simulink model "decimation_fir"  (Simulink 7.3)
settings: Solver=FixedStepDiscrete  StartTime=0.0  StopTime=3000 * SampleTime  RelTol=1e-3
PreLoadFcn:
  | setup_decimation_fir;
InitFcn:
  | setup_decimation_fir;
values from neighbouring files (symbols this model uses):
  ChanCycleCount = ceil(ChanCount/ChanWireCount)    [setup_decimation_fir.m]
  ChanWireCount = ceil(ChanCount/Period)    [setup_decimation_fir.m]
  ClockRate = ' num2str(ClockRate) '    [setup_decimation_fir.m]
  Period = ClockRate / SampleRate    (= 4)    [setup_decimation_fir.m]
  period_out = Period*Decimation    (= 16)    [setup_decimation_fir.m]
  SampleTime = 1    [setup_decimation_fir.m]
libraries: DSPBABase x8, simulink x7, dspsrcs4 x2
Description:
  | This model shows how to use the DecimatingFIR block to build a 16-channel decimate by 5 49-tap FIR filter. The target system clock frequency is 240 MHz.
  | The model will generate RTL that can be used in the third party tools.
  | The parameters for the system can be modified in the file setup_demo_fird.m which can be accessed from the Edit Params icon.
settings Model: Creator=sichou  LastModifiedBy=xdong
settings OptimizationCC: InitFltsAndDblsToZero=on
settings DebuggingCC: SaveWithParameterizedLinksMsg=none  SignalResolutionControl=TryResolveAllWithWarning  MultiTaskDSMMsg=warning  MultiTaskCondExecSysMsg=none  StrictBusMsg=None
settings RTWCC: IncludeERTFirstTime=on
settings GRTTargetCC: TargetFcnLib=ansi_tfl_tmw.mat

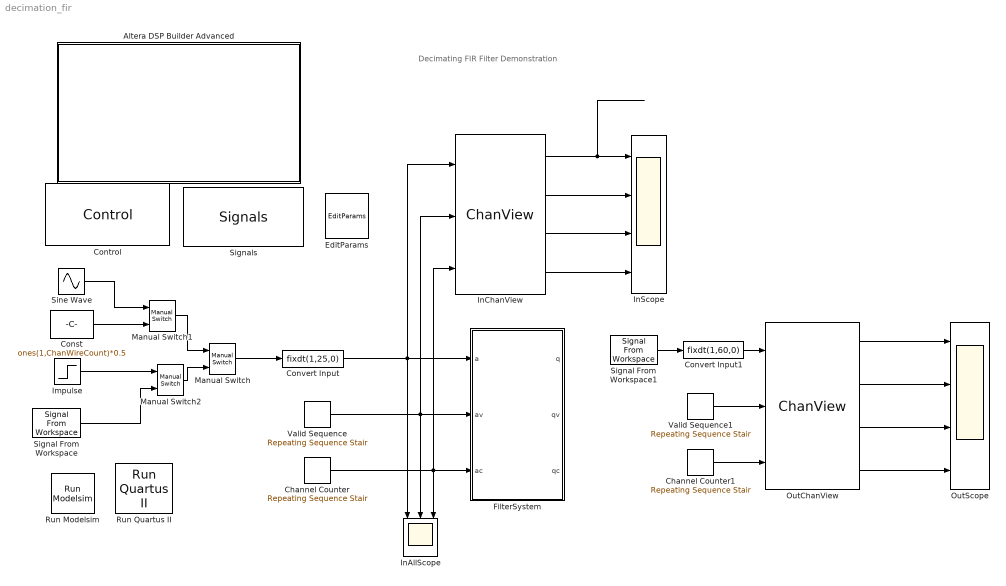
== system decimation_fir ==
  note: Decimating FIR Filter Demonstration
  Altera DSP Builder Advanced : Subsystem
      settings: OpenFcn=web('http://www.altera.com', '-new');
      mask Type: DSP Builder Advanced Blockset Ignored Block
      mask Display: image(imread('alteralogo.tif'));
  Channel Counter : simulink/Sources/Repeating Sequence Stair  SystemSampleTime=-1  OutValues=[0:ChanCycleCount-1 zeros(1,Period-ChanCycleCount)]  tsamp=SampleTime  OutMin=[]  OutMax=[]  OutDataTypeStr=uint(8)  OutputDataTypeScalingMode=Specify via dialog  OutDataType=uint(8)  ConRadixGroup=Best Precision: Vector-wise  OutScaling=2^-12
  Channel Counter1 : simulink/Sources/Repeating Sequence Stair  SystemSampleTime=-1  OutValues=0:ChanCycleCount-1 %[0:ChanCycleCount-1 zeros(1,period_out-ChanCycleCount)]  tsamp=SampleTime  OutMin=[]  OutMax=[]  OutDataTypeStr=uint(8)  OutputDataTypeScalingMode=Specify via dialog  OutDataType=uint(8)  ConRadixGroup=Best Precision: Vector-wise  OutScaling=2^-12
  Const : Constant  Value=ones(1,ChanWireCount)*0.5  OutDataType=sfix(16)  OutScaling=2^0
  Control : DSPBABase/Control  generate=off  destination=../rtl  language=VHDL  autotestbench=on  signaldepth=2  coveragetestbench=off  logs=off  spacewidth=2  spacenum=2  addrwidth=11  datawidth=16  dataendian=Big Endian  hierarchicalnames=on  ramThresholdBits=-1  distRamThresholdBits=-1  mlabThresholdBits=-1  hardMultiplierThresholdLuts=-1  version=20090407
  Convert Input : DataTypeConversion  OutDataTypeMode=Specify via dialog  OutDataType=fixdt(1,25,0)  OutDataTypeStr=fixdt(1,25,0)  SaturateOnIntegerOverflow=on
  Convert Input1 : DataTypeConversion  OutDataTypeMode=Specify via dialog  OutDataType=fixdt(1,60,0)  OutDataTypeStr=fixdt(1,60,0)  SaturateOnIntegerOverflow=on
  EditParams : DSPBABase/EditParams  SystemSampleTime=-1  version=20090407
  FilterSystem : Subsystem
  Impulse : Step  Time=ones(1, ChanWireCount)  Before=1  After=0  SampleTime=SampleTime
  InAllScope : Scope  NumInputPorts=3
      settings: TimeRange=2000  YMin=0~0.95~-1  YMax=20~1.05~1  SaveName=ScopeData4
  InChanView : DSPBABase/ChanView  nchans=ChanCount  chan_vector=[0:3]  latency=0  version=20090407
  InScope : Scope  NumInputPorts=4
      settings: TimeRange=1.745762711864407e-005  YMin=-1~-1~-1~-1  YMax=1~1~1~1  SaveName=ScopeData6
  Manual Switch : simulink/Signal Routing/Manual Switch  SystemSampleTime=-1  sw=0  action=0  varsize=off
  Manual Switch1 : simulink/Signal Routing/Manual Switch  SystemSampleTime=-1  sw=1  action=0  varsize=off
  Manual Switch2 : simulink/Signal Routing/Manual Switch  SystemSampleTime=-1  sw=0  action=0  varsize=off
  OutChanView : DSPBABase/ChanView  nchans=ChanCount  chan_vector=[0 1 2 3]  latency=0  version=20090407
  OutScope : Scope  NumInputPorts=4
      settings: TimeRange=1.920415224913495e-005  YMin=-0.5~-0.5~-0.5~-0.5  YMax=0.5~0.5~0.5~0.5  SaveName=ScopeData5
  Run Modelsim : DSPBABase/Run Modelsim  SystemSampleTime=-1  version=20090407
  Run Quartus II : DSPBABase/Run Quartus II  SystemSampleTime=-1  version=20090407
  Signal From Workspace : dspsrcs4/Signal From Workspace  SystemSampleTime=-1  X=sine_decimation_fir_input  Ts=1  nsamps=1  OutputAfterFinalValue=Setting to zero  ignoreOrWarnInputAndFrameLengths=off
  Signal From Workspace1 : dspsrcs4/Signal From Workspace  SystemSampleTime=-1  X=dout  Ts=1  nsamps=1  OutputAfterFinalValue=Setting to zero  ignoreOrWarnInputAndFrameLengths=off
  Signals : DSPBABase/Signals  SystemSampleTime=-1  clk=clk  freq=ClockRate  margin=ClockMargin  rst=areset  rstactive=High  bus=bus  enbusclock=on  busfreq=ClockRate / 4  bussync=on  version=20090407
  Sine Wave : Sin  SineType=Sample based  Amplitude=ones(1,ChanWireCount)*(2^17-2)/(2^17)  Bias=0  Frequency=(2 * pi) / ( 4 * 2^24 / floor(2^24 * 0.051))  Phase=0  Samples=500  SampleTime=SampleTime  Offset=0
  Valid Sequence : simulink/Sources/Repeating Sequence Stair  SystemSampleTime=-1  OutValues=[ones(1,ChanCycleCount) zeros(1,Period-ChanCycleCount)]  tsamp=SampleTime  OutMin=[]  OutMax=[]  OutDataTypeStr=Inherit: Inherit via back propagation  OutDataType=float('double')  ConRadixGroup=Best Precision: Vector-wise  OutScaling=2^-12
  Valid Sequence1 : simulink/Sources/Repeating Sequence Stair  SystemSampleTime=-1  OutValues=ones(1, ChanCycleCount) %[ones(1,ChanCycleCount) zeros(1,period_out-ChanCycleCount)]  tsamp=SampleTime  OutMin=[]  OutMax=[]  OutDataTypeStr=Inherit: Inherit via back propagation  OutDataType=float('double')  ConRadixGroup=Best Precision: Vector-wise  OutScaling=2^-12
  wires:
  Channel Counter/1 -> InChanView/3, FilterSystem/3(ac), InAllScope/3
  Manual Switch2/1 -> Manual Switch/2
  Impulse/1 -> Manual Switch2/1
  Valid Sequence/1 -> FilterSystem/2(av), InChanView/2, InAllScope/2
  OutChanView/1 -> OutScope/1
  OutChanView/2 -> OutScope/2
  OutChanView/3 -> OutScope/3
  OutChanView/4 -> OutScope/4
  Signal From Workspace/1 -> Manual Switch2/2
  InChanView/1 -> InScope/1
  InChanView/2 -> InScope/2
  InChanView/3 -> InScope/3
  InChanView/4 -> InScope/4
  Manual Switch/1 -> Convert Input/1
  Convert Input/1 -> FilterSystem/1(a), InChanView/1, InAllScope/1
  Sine Wave/1 -> Manual Switch1/1
  Const/1 -> Manual Switch1/2
  Manual Switch1/1 -> Manual Switch/1
  Valid Sequence1/1 -> OutChanView/2
  Channel Counter1/1 -> OutChanView/3
  Signal From Workspace1/1 -> Convert Input1/1
  Convert Input1/1 -> OutChanView/1

== system decimation_fir/Altera DSP Builder Advanced ==

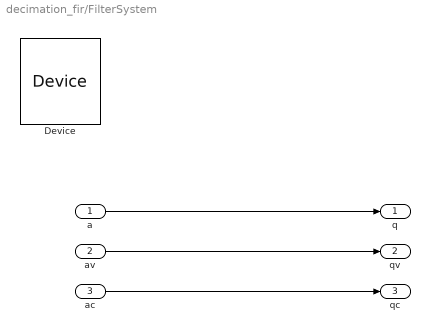
== system decimation_fir/FilterSystem ==
  a : Inport  OutDataType=sfix(16)  OutScaling=2^0
  av : Inport  Port=2  OutDataType=sfix(16)  OutScaling=2^0
  ac : Inport  Port=3  OutDataType=sfix(16)  OutScaling=2^0
  Device : DSPBABase/Device  SystemSampleTime=-1  family=Stratix II  stratix4device=Stratix IV E  hardcopy4device=HardCopy IV E  device=AUTO  speed=-3  stratixSpeed=-5  stratix2Speed=-3  stratix3Speed=-2  stratix4gxSpeed=-2  stratix4gtSpeed=-1  cyclone2Speed=-6  cyclone3Speed=-6  arria2Speed=-4  ecp2Speed=-7  version=20090914
  q : Outport  OutDataType=sfix(16)  OutScaling=2^0
  qv : Outport  Port=2  OutDataType=sfix(16)  OutScaling=2^0
  qc : Outport  Port=3  OutDataType=sfix(16)  OutScaling=2^0
  wires:
  a/1 -> q/1
  ac/1 -> qc/1
  av/1 -> qv/1
